simulink model "ArduinoDue"  (R2013a)
settings: Solver=FixedStepDiscrete  StartTime=0.0  StopTime=inf  FixedStep=0.008  RelTol=1e-3
libraries: simulink x2, qbmove_library x2, QB_pacer_lib x1
settings Model: Creator=laurentio  LastModifiedBy=Marco

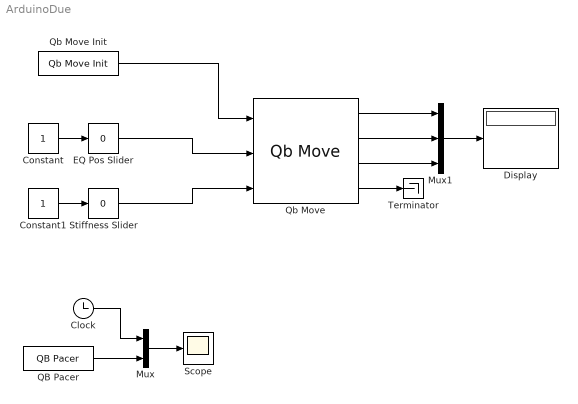
== system ArduinoDue ==
  Clock : Clock
  Constant : Constant
  Constant1 : Constant
  Display : Display
  "EQ Pos Slider " : simulink/Math Operations/Slider Gain  low=-180  gain=0  high=180
  Mux : Mux  Inputs=2
  Mux1 : Mux  Inputs=3
  QB Pacer : QB_pacer_lib/QB Pacer  simTimePerRealTime=1
  Qb Move : qbmove_library/Qb Move  ID=2  ACTIVE_COMM_DIRECTIONS=Both  CONTROL_MODE=Equilibrium Position and Stiffness Preset  DAISY_CHAINING=off  MAX_ANG=0  SW_LIMIT=inf  OFFSET=0
  Qb Move Init : qbmove_library/Qb Move Init  NUMBER_OF_COM='COM1'  BAUD_RATE_COM=115200
  Scope : Scope
      settings: YMin=0  YMax=5.5
  Stiffness Slider : simulink/Math Operations/Slider Gain  low=0  gain=0  high=35
  Terminator : Terminator
  wires:
  Qb Move Init/1 -> Qb Move/1
  Constant/1 -> "EQ Pos Slider "/1
  "EQ Pos Slider "/1 -> Qb Move/2
  Constant1/1 -> Stiffness Slider/1
  Stiffness Slider/1 -> Qb Move/3
  QB Pacer/1 -> Mux/2
  Clock/1 -> Mux/1
  Mux/1 -> Scope/1
  Qb Move/1 -> Mux1/1
  Qb Move/2 -> Mux1/2
  Qb Move/3 -> Mux1/3
  Qb Move/4 -> Terminator/1
  Mux1/1 -> Display/1
